simulink library "VIS_LIB"  (Simulink 8.6)
settings: Solver=ode45  StartTime=0.0  StopTime=10.0  RelTol=1e-3
undefined symbols (not defined in the file): AC, SIXOSEM_F_WD_AC_MASTER
libraries: cdsFilt x376, cdsEpicsOut x253, cdsEpicsIn x179, cdsTP x123, VIS_LIB x95, cdsMuxMatrix x91, cdsEpicsStringIn x75, cdsFiltCtrl x72, cdsFunctionCall x70, cdsRms x59, KAGRA_UTIL x25, STATE_BIO_MASTER x5
(part 1 of 38)
settings Model: Creator=keiko  LastModifiedBy=controls

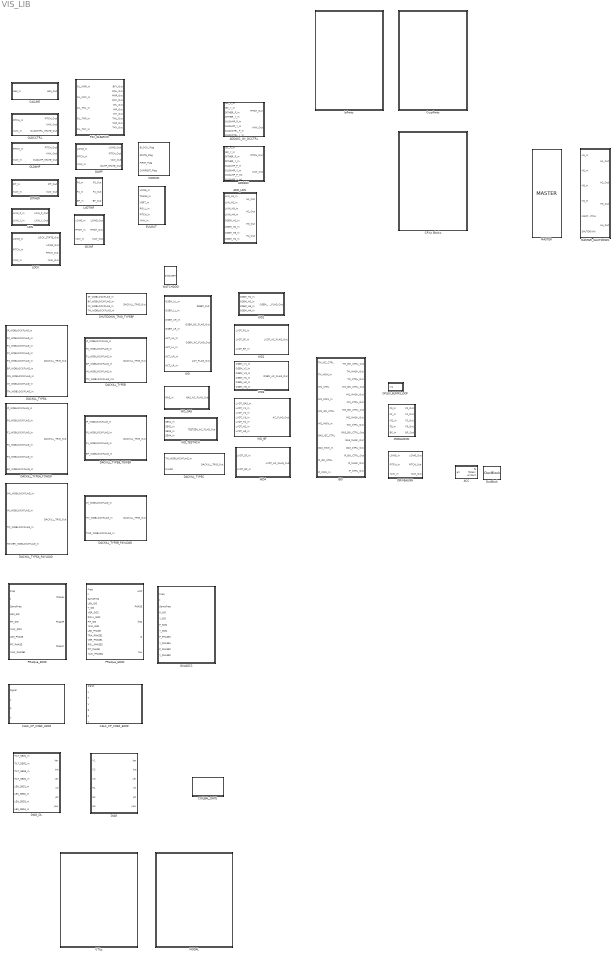
== system VIS_LIB ==
  ACC : Subsystem
  ADDASC : Subsystem
  ADDASC_W/_DCCTRL : Subsystem
  ADD_LKIN : Subsystem
  BIO : Subsystem
  CALC_CP_COEF_3DOF : Subsystem
  CALC_CP_COEF_6DOF : Subsystem
  CALLINE : Subsystem
  COILBAL_DATE : Subsystem
  CRYp Blocks : Subsystem
  CrypParts : Subsystem
  DACKILL_TYPEA : Subsystem
  DACKILL_TYPEA_PAYLOAD : Subsystem
  DACKILL_TYPEA_TOWER : Subsystem
  DACKILL_TYPEB : Subsystem
  DACKILL_TYPEB_PAYLOAD : Subsystem
  DACKILL_TYPEB_TOWER : Subsystem
  "DACKILL_TYPEC " : Subsystem
  DAMP : Subsystem
  DIAG : Subsystem
  DIAG_OL : Subsystem
  DITHER : Subsystem
  DRIVEALIGN : Subsystem
  DocBlock : simulink/Model-Wide Utilities/DocBlock  DocumentType=Text
  EULOUT : Subsystem
  ISCINF : Subsystem
  IpParts : Subsystem
  LKIN : Subsystem
  LOCK : Subsystem
  LVDTINF : Subsystem
  MASTER : CRYP_TM_MASTER/CRYP_TM_MASTER/MASTER
  MASTER_SHUTDOWN : Subsystem
  MODAL : Subsystem
  MODALMON : Subsystem
  OLDAMP : Subsystem
  OLDCCTRL : Subsystem
  OPLEV_BLRMS_DOF : Subsystem
  PAY_OLSERVO : Subsystem
  PReQua_3DOF : Subsystem
  PReQua_6DOF : Subsystem
  QUAASC1 : Subsystem
  SHUTDOWN_TRIG_TYPEBP : Subsystem
  UTILs : Subsystem
  WATCHDOG : cdsFunctionCall/Subsystem  Tag=cdsFunctionCall  Description=inline OSEMWATCHDOG $SUS_SRC/WATCHDOG.c
      settings: AttributesFormatString=%<Tag>\n%<Description>
  WD : Subsystem
  WD1 : Subsystem
  WD2 : Subsystem
  WD3 : Subsystem
  WD4 : Subsystem  AncestorBlock=VIS_LIB/WD2
  WDMON : Subsystem
  WD_BF : Subsystem
  WD_GAS : Subsystem
  WD_TEST4CH : Subsystem

== system VIS_LIB/ACC ==
  note: #DAQ Channels
      |
      | ACCSERVO_IN1 2048
      | ACCSERVO_OUT 2048
      | ERR2ACC_OUT 2048
      | FB2ACC_OUT 2048
  err : Inport
  ACCSERVO : cdsFilt/Subsystem  Tag=cdsFilt  Description=|
      | Purpose:                                                                                                                                                                                                                                  
      | Standard CDS IIR filter module.                                                                                                                                                                                                           
      |                                                                                                                                                                                                                                           
      | Operation:                                                                                                                                                                                                                                
      | Consists of 10 second order section IIR filters, plus a ramped gain stage. In FE code, also provides pre-defined test points and excitation channel inputs. The filter coefficients are defined in the LIGO system using the 'foton' tool.
      |                                                                                                                                                                                                                                           
      | Usage:                                                                                                                                                                                                                                    
      | Name the part with the desired filter module name.
      settings: AttributesFormatString=%<Tag>
  ERR2ACC : cdsFilt/Subsystem  Tag=cdsFilt  Description=|
      | Purpose:                                                                                                                                                                                                                                  
      | Standard CDS IIR filter module.                                                                                                                                                                                                           
      |                                                                                                                                                                                                                                           
      | Operation:                                                                                                                                                                                                                                
      | Consists of 10 second order section IIR filters, plus a ramped gain stage. In FE code, also provides pre-defined test points and excitation channel inputs. The filter coefficients are defined in the LIGO system using the 'foton' tool.
      |                                                                                                                                                                                                                                           
      | Usage:                                                                                                                                                                                                                                    
      | Name the part with the desired filter module name.
      settings: AttributesFormatString=%<Tag>
  FB2ACC : cdsFilt/Subsystem  Tag=cdsFilt  Description=|
      | Purpose:                                                                                                                                                                                                                                  
      | Standard CDS IIR filter module.                                                                                                                                                                                                           
      |                                                                                                                                                                                                                                           
      | Operation:                                                                                                                                                                                                                                
      | Consists of 10 second order section IIR filters, plus a ramped gain stage. In FE code, also provides pre-defined test points and excitation channel inputs. The filter coefficients are defined in the LIGO system using the 'foton' tool.
      |                                                                                                                                                                                                                                           
      | Usage:                                                                                                                                                                                                                                    
      | Name the part with the desired filter module name.
      settings: AttributesFormatString=%<Tag>
  fb : Outport
  fb2acc : Outport  Port=2
  err2acc : Outport  Port=3
  wires:
  ERR2ACC/1 -> err2acc/1
  FB2ACC/1 -> fb2acc/1
  ACCSERVO/1 -> FB2ACC/1, fb/1
  err/1 -> ACCSERVO/1, ERR2ACC/1

== system VIS_LIB/ADDASC ==
  ISC_P_In : Inport
  ISC_Y_In : Inport  Port=2
  DITHER_P_In : Inport  Port=3
  DITHER_Y_In : Inport  Port=4
  OLDAMP_P_In : Inport  Port=5
  OLDAMP_Y_In : Inport  Port=6
  OLDAMP_P_In2 : Inport  Port=7
  OLDAMP_Y_In1 : Inport  Port=8
  Sum3 : Sum  Inputs=++++
  Sum4 : Sum  Inputs=++++
  PITCH_Out : Outport
  YAW_Out : Outport  Port=2
  wires:
  DITHER_Y_In/1 -> Sum3/2
  DITHER_P_In/1 -> Sum4/2
  Sum4/1 -> PITCH_Out/1
  ISC_Y_In/1 -> Sum3/1
  ISC_P_In/1 -> Sum4/1
  Sum3/1 -> YAW_Out/1
  OLDAMP_P_In/1 -> Sum4/3
  OLDAMP_Y_In/1 -> Sum3/3
  OLDAMP_P_In2/1 -> Sum4/4
  OLDAMP_Y_In1/1 -> Sum3/4

== system VIS_LIB/ADDASC_W/_DCCTRL ==
  ISC_P_In : Inport
  ISC_Y_In : Inport  Port=2
  DITHER_P_In : Inport  Port=3
  DITHER_Y_In : Inport  Port=4
  OLDAMP_P_In : Inport  Port=5
  OLDAMP_Y_In : Inport  Port=6
  OLDCCTRL_P_In : Inport  Port=7
  OLDCCTRL_Y_In : Inport  Port=8
  Sum3 : Sum  Inputs=++++
  Sum4 : Sum  Inputs=++++
  PITCH_Out : Outport
  YAW_Out : Outport  Port=2
  wires:
  OLDAMP_Y_In/1 -> Sum3/3
  DITHER_Y_In/1 -> Sum3/2
  DITHER_P_In/1 -> Sum4/2
  OLDAMP_P_In/1 -> Sum4/3
  Sum4/1 -> PITCH_Out/1
  ISC_Y_In/1 -> Sum3/1
  ISC_P_In/1 -> Sum4/1
  Sum3/1 -> YAW_Out/1
  OLDCCTRL_P_In/1 -> Sum4/4
  OLDCCTRL_Y_In/1 -> Sum3/4

== system VIS_LIB/ADD_LKIN ==
  LKN_H1_In : Inport
  LKN_H2_In : Inport  Port=2
  LKIN_H3_In : Inport  Port=3
  LKIN_H4_In : Inport  Port=4
  OSEM_H1_In : Inport  Port=5
  OSEM_H2_In : Inport  Port=6
  OSEM_H3_In : Inport  Port=7
  OSEM_H4_In : Inport  Port=8
  Sum{,1,3..4} (4 alike) : Sum
  H1_Out : Outport
  H2_Out : Outport  Port=2
  H3_Out : Outport  Port=3
  H4_Out : Outport  Port=4
  wires:
  LKIN_H4_In/1 -> Sum1/1
  LKIN_H3_In/1 -> Sum3/1
  LKN_H2_In/1 -> Sum4/1
  Sum/1 -> H1_Out/1
  LKN_H1_In/1 -> Sum/1
  OSEM_H1_In/1 -> Sum/2
  Sum3/1 -> H3_Out/1
  Sum4/1 -> H2_Out/1
  OSEM_H3_In/1 -> Sum3/2
  OSEM_H2_In/1 -> Sum4/2
  Sum1/1 -> H4_Out/1
  OSEM_H4_In/1 -> Sum1/2

== system VIS_LIB/BIO ==
  note: 12 Bit Word
  note: 12 Bit Word
  note: 12 Bit Word
  note: 12 Bit Word
  TM_ISC_CTRL : Inport
  TM_MON_In : Inport  Port=2
  IM1_CTRL : Inport  Port=3
  IM1_MON_In : Inport  Port=4
  IM2_ISC_CTRL : Inport  Port=5
  IM2_MON_In : Inport  Port=6
  GAS_ISC_CTRL : Inport  Port=7
  GAS_MON_In : Inport  Port=8
  IP_ISC_CTRL : Inport  Port=9
  IP_MON_In : Inport  Port=10
  GAS : STATE_BIO_MASTER/UIM_BIO_MASTER
  IM1 : STATE_BIO_MASTER/UIM_BIO_MASTER
  IM2 : STATE_BIO_MASTER/UIM_BIO_MASTER
  IP : STATE_BIO_MASTER/TACQ_BIO_MASTER
  TM : STATE_BIO_MASTER/UIM_BIO_MASTER
  TM_BO_CTRL_Out : Outport
  TM_MASK_Out : Outport  Port=2
  TM_CTRL_Out : Outport  Port=3
  IM1_BO_CTRL_Out : Outport  Port=4
  IM1_MASK_Out : Outport  Port=5
  IM1_CTRL_Out : Outport  Port=6
  IM2_BO_CTRL_Out : Outport  Port=7
  IM2_MASK_Out : Outport  Port=8
  IM2_CTRL_Out : Outport  Port=9
  GAS_BO_CTRL_Out : Outport  Port=10
  GAS_MASK_Out : Outport  Port=11
  GAS_CTRL_Out : Outport  Port=12
  IP_BO_CTRL_Out : Outport  Port=13
  IP_MASK_Out : Outport  Port=14
  IP_CTRL_Out : Outport  Port=15
  wires:
  IP/3 -> IP_BO_CTRL_Out/1
  IP/2 -> IP_CTRL_Out/1
  IP/1 -> IP_MASK_Out/1
  GAS/3 -> GAS_BO_CTRL_Out/1
  GAS/2 -> GAS_CTRL_Out/1
  GAS/1 -> GAS_MASK_Out/1
  IM2/3 -> IM2_BO_CTRL_Out/1
  IM2/2 -> IM2_CTRL_Out/1
  IM2/1 -> IM2_MASK_Out/1
  IM1/3 -> IM1_BO_CTRL_Out/1
  IM1/2 -> IM1_CTRL_Out/1
  IM1/1 -> IM1_MASK_Out/1
  TM/3 -> TM_BO_CTRL_Out/1
  TM/2 -> TM_CTRL_Out/1
  TM/1 -> TM_MASK_Out/1
  IP_ISC_CTRL/1 -> IP/1
  IP_MON_In/1 -> IP/2
  GAS_ISC_CTRL/1 -> GAS/1
  GAS_MON_In/1 -> GAS/2
  IM2_ISC_CTRL/1 -> IM2/1
  IM2_MON_In/1 -> IM2/2
  IM1_MON_In/1 -> IM1/2
  IM1_CTRL/1 -> IM1/1
  TM_ISC_CTRL/1 -> TM/1
  TM_MON_In/1 -> TM/2

== system VIS_LIB/CALC_CP_COEF_3DOF ==
  Signal : Inport
  L : Inport  Port=2
  P : Inport  Port=3
  Y : Inport  Port=4
  BASE_SLCT : cdsMuxMatrix/Subsystem  Tag=cdsMuxMatrix  Description=Any size matrix. Inputs and outputs must be connected using Mux and Demux parts.
      settings: AttributesFormatString=%<Tag>
  COEF : cdsFilt/Subsystem  Tag=cdsFilt  Description=|
      | Purpose:                                                                                                                                                                                                                                  
      | Standard CDS IIR filter module.                                                                                                                                                                                                           
      |                                                                                                                                                                                                                                           
      | Operation:                                                                                                                                                                                                                                
      | Consists of 10 second order section IIR filters, plus a ramped gain stage. In FE code, also provides pre-defined test points and excitation channel inputs. The filter coefficients are defined in the LIGO system using the 'foton' tool.
      |                                                                                                                                                                                                                                           
      | Usage:                                                                                                                                                                                                                                    
      | Name the part with the desired filter module name.
      settings: AttributesFormatString=%<Tag>
  Demux1 : Demux  Outputs=1
  Divide : Product  Inputs=*/
  Mux1 : Mux  Inputs=3
  Terminator3 : Terminator
  wires:
  Y/1 -> Mux1/3
  BASE_SLCT/1 -> Demux1/1
  L/1 -> Mux1/1
  Demux1/1 -> Divide/2
  COEF/1 -> Terminator3/1
  Mux1/1 -> BASE_SLCT/1
  Signal/1 -> Divide/1
  Divide/1 -> COEF/1
  P/1 -> Mux1/2

== system VIS_LIB/CALC_CP_COEF_6DOF ==
  Signal : Inport
  L : Inport  Port=2
  T : Inport  Port=3
  V : Inport  Port=4
  R : Inport  Port=5
  P : Inport  Port=6
  Y : Inport  Port=7
  BASE_SLCT : cdsMuxMatrix/Subsystem  Tag=cdsMuxMatrix  Description=Any size matrix. Inputs and outputs must be connected using Mux and Demux parts.
      settings: AttributesFormatString=%<Tag>
  COEF : cdsFilt/Subsystem  Tag=cdsFilt  Description=|
      | Purpose:                                                                                                                                                                                                                                  
      | Standard CDS IIR filter module.                                                                                                                                                                                                           
      |                                                                                                                                                                                                                                           
      | Operation:                                                                                                                                                                                                                                
      | Consists of 10 second order section IIR filters, plus a ramped gain stage. In FE code, also provides pre-defined test points and excitation channel inputs. The filter coefficients are defined in the LIGO system using the 'foton' tool.
      |                                                                                                                                                                                                                                           
      | Usage:                                                                                                                                                                                                                                    
      | Name the part with the desired filter module name.
      settings: AttributesFormatString=%<Tag>
  Demux1 : Demux  Outputs=1
  Divide : Product  Inputs=*/
  Mux1 : Mux  Inputs=6
  wires:
  Divide/1 -> COEF/1
  Signal/1 -> Divide/1
  Mux1/1 -> BASE_SLCT/1
  Demux1/1 -> Divide/2
  BASE_SLCT/1 -> Demux1/1
  L/1 -> Mux1/1
  T/1 -> Mux1/2
  V/1 -> Mux1/3
  R/1 -> Mux1/4
  P/1 -> Mux1/5
  Y/1 -> Mux1/6

== system VIS_LIB/CALLINE ==
  LEN_In : Inport
  L : cdsFilt/Subsystem  Tag=cdsFilt  Description=|
      | Purpose:                                                                                                                                                                                                                                  
      | Standard CDS IIR filter module.                                                                                                                                                                                                           
      |                                                                                                                                                                                                                                           
      | Operation:                                                                                                                                                                                                                                
      | Consists of 10 second order section IIR filters, plus a ramped gain stage. In FE code, also provides pre-defined test points and excitation channel inputs. The filter coefficients are defined in the LIGO system using the 'foton' tool.
      |                                                                                                                                                                                                                                           
      | Usage:                                                                                                                                                                                                                                    
      | Name the part with the desired filter module name.
      settings: AttributesFormatString=%<Tag>
  LEN_Out : Outport
  wires:
  LEN_In/1 -> L/1
  L/1 -> LEN_Out/1

== system VIS_LIB/COILBAL_DATE ==
  DAY : cdsEpicsIn/Subsystem  Tag=cdsEpicsIn  Description=|
      | Purpose:                                                                              
      | Create an EPICS input channel connection to the FE realtime controls.                 
      |                                                                                       
      | Operation:                                                                            
      | Outputs value from an EPICS ai record. Value is floating point with a precision of 3..
      |                                                                                       
      | Usage:                                                                                
      | Name the part with the desired EPICS channel name.
      settings: AttributesFormatString=%<Tag>
  HOUR : cdsEpicsIn/Subsystem  Tag=cdsEpicsIn  Description=|
      | Purpose:                                                                              
      | Create an EPICS input channel connection to the FE realtime controls.                 
      |                                                                                       
      | Operation:                                                                            
      | Outputs value from an EPICS ai record. Value is floating point with a precision of 3..
      |                                                                                       
      | Usage:                                                                                
      | Name the part with the desired EPICS channel name.
      settings: AttributesFormatString=%<Tag>
  MIN : cdsEpicsIn/Subsystem  Tag=cdsEpicsIn  Description=|
      | Purpose:                                                                              
      | Create an EPICS input channel connection to the FE realtime controls.                 
      |                                                                                       
      | Operation:                                                                            
      | Outputs value from an EPICS ai record. Value is floating point with a precision of 3..
      |                                                                                       
      | Usage:                                                                                
      | Name the part with the desired EPICS channel name.
      settings: AttributesFormatString=%<Tag>
  MON : cdsEpicsIn/Subsystem  Tag=cdsEpicsIn  Description=|
      | Purpose:                                                                              
      | Create an EPICS input channel connection to the FE realtime controls.                 
      |                                                                                       
      | Operation:                                                                            
      | Outputs value from an EPICS ai record. Value is floating point with a precision of 3..
      |                                                                                       
      | Usage:                                                                                
      | Name the part with the desired EPICS channel name.
      settings: AttributesFormatString=%<Tag>
  Terminator{1..5} (5 alike) : Terminator
  YEAR : cdsEpicsIn/Subsystem  Tag=cdsEpicsIn  Description=|
      | Purpose:                                                                              
      | Create an EPICS input channel connection to the FE realtime controls.                 
      |                                                                                       
      | Operation:                                                                            
      | Outputs value from an EPICS ai record. Value is floating point with a precision of 3..
      |                                                                                       
      | Usage:                                                                                
      | Name the part with the desired EPICS channel name.
      settings: AttributesFormatString=%<Tag>
  wires:
  MIN/1 -> Terminator5/1
  DAY/1 -> Terminator3/1
  HOUR/1 -> Terminator4/1
  MON/1 -> Terminator2/1
  YEAR/1 -> Terminator1/1

== system VIS_LIB/CRYp Blocks ==
  COILOUTF : Subsystem
  MASTER : Subsystem
  PSWD : Subsystem

== system VIS_LIB/CrypParts ==
  ADD : Subsystem
  ADDALL : Subsystem
  ADDISC_IM : Subsystem
  ADDISC_MN : Subsystem
  ADDLOCAL_IM : Subsystem
  ADDLOCAL_MN : Subsystem
  ADD_TM : Subsystem
  DAMP : Subsystem
  DAMP_PY : Subsystem
  DRIVEALIGN : Subsystem
  LOCK : Subsystem
  OLDCCTRL : Subsystem
  OPLEV : Subsystem
  OPTICALIGN : Subsystem
  PSDAMP : Subsystem
  PSINF : Subsystem
  SUMOUT : Subsystem
  SUMOUT_TM : Subsystem
  TEST : Subsystem
  TEST_TM : Subsystem
  TM_OLSET : Subsystem

== system VIS_LIB/DACKILL_TYPEA ==
  note: WDBLOCKFLAG is zero (0) if OK,
      | non-zero if BAD
  note: AND is zero  (0) if all stages are OK
      | non-zero if BAD
  IP_WDBLOCKFLAG_In : Inport
  F0_WDBLOCKFLAG_In : Inport  Port=2
  F1_WDBLOCKFLAG_In : Inport  Port=3
  F2_WDBLOCKFLAG_In : Inport  Port=4
  F3_WDBLOCKFLAG_In : Inport  Port=5
  BF_WDBLOCKFLAG_In : Inport  Port=6
  MN_WDBLOCKFLAG_In : Inport  Port=7
  IM_WDBLOCKFLAG_In : Inport  Port=8
  TM_WDBLOCKFLAG_In : Inport  Port=9
  LogicalOperator1 : Logic  Operator=OR  Inputs=9  AllPortsSameDT=off  OutDataTypeStr=boolean
  STATE : cdsEpicsOut/Subsystem  Tag=cdsEpicsOutput  Description=|
      | Purpose:                                          
      | Output a FE signal to an EPICS channel.           
      |                                                   
      | Operation:                                        
      | Takes input value and passes it to EPICS record.  
      |                                                   
      | Usage:                                            
      | Name the part with the desired EPICS rrecord name.
      settings: AttributesFormatString=%<Tag>
  DACKILL_TRIG_Out : Outport
  wires:
  STATE/1 -> DACKILL_TRIG_Out/1
  IP_WDBLOCKFLAG_In/1 -> LogicalOperator1/1
  F0_WDBLOCKFLAG_In/1 -> LogicalOperator1/2
  F1_WDBLOCKFLAG_In/1 -> LogicalOperator1/3
  LogicalOperator1/1 -> STATE/1
  IM_WDBLOCKFLAG_In/1 -> LogicalOperator1/8
  BF_WDBLOCKFLAG_In/1 -> LogicalOperator1/6
  TM_WDBLOCKFLAG_In/1 -> LogicalOperator1/9
  MN_WDBLOCKFLAG_In/1 -> LogicalOperator1/7
  F3_WDBLOCKFLAG_In/1 -> LogicalOperator1/5
  F2_WDBLOCKFLAG_In/1 -> LogicalOperator1/4

== system VIS_LIB/DACKILL_TYPEA_PAYLOAD ==
  note: WDBLOCKFLAG is zero (0) if OK,
      | non-zero if BAD
  note: AND is zero  (0) if all stages are OK
      | non-zero if BAD
  MN_WDBLOCKFLAG_In : Inport
  IM_WDBLOCKFLAG_In : Inport  Port=2
  TM_WDBLOCKFLAG_In : Inport  Port=3
  TOWER_WDBLOCKFLAG_In : Inport  Port=4
  LogicalOperator1 : Logic  Operator=OR  Inputs=3  AllPortsSameDT=off  OutDataTypeStr=boolean
  LogicalOperator2 : Logic  Operator=OR  AllPortsSameDT=off  OutDataTypeStr=boolean
  PAYLOAD_STATE : cdsEpicsOut/Subsystem  Tag=cdsEpicsOutput  Description=|
      | Purpose:                                          
      | Output a FE signal to an EPICS channel.           
      |                                                   
      | Operation:                                        
      | Takes input value and passes it to EPICS record.  
      |                                                   
      | Usage:                                            
      | Name the part with the desired EPICS rrecord name.
      settings: AttributesFormatString=%<Tag>
  STATE : cdsEpicsOut/Subsystem  Tag=cdsEpicsOutput  Description=|
      | Purpose:                                          
      | Output a FE signal to an EPICS channel.           
      |                                                   
      | Operation:                                        
      | Takes input value and passes it to EPICS record.  
      |                                                   
      | Usage:                                            
      | Name the part with the desired EPICS rrecord name.
      settings: AttributesFormatString=%<Tag>
  DACKILL_TRIG_Out : Outport
  wires:
  LogicalOperator1/1 -> PAYLOAD_STATE/1
  IM_WDBLOCKFLAG_In/1 -> LogicalOperator1/2
  TM_WDBLOCKFLAG_In/1 -> LogicalOperator1/3
  MN_WDBLOCKFLAG_In/1 -> LogicalOperator1/1
  TOWER_WDBLOCKFLAG_In/1 -> LogicalOperator2/2
  PAYLOAD_STATE/1 -> LogicalOperator2/1
  LogicalOperator2/1 -> STATE/1
  STATE/1 -> DACKILL_TRIG_Out/1

== system VIS_LIB/DACKILL_TYPEA_TOWER ==
  note: WDBLOCKFLAG is zero (0) if OK,
      | non-zero if BAD
  note: AND is zero  (0) if all stages are OK
      | non-zero if BAD
  IP_WDBLOCKFLAG_In : Inport
  F0_WDBLOCKFLAG_In : Inport  Port=2
  F1_WDBLOCKFLAG_In : Inport  Port=3
  F2_WDBLOCKFLAG_In : Inport  Port=4
  F3_WDBLOCKFLAG_In : Inport  Port=5
  BF_WDBLOCKFLAG_In : Inport  Port=6
  LogicalOperator1 : Logic  Operator=OR  Inputs=6  AllPortsSameDT=off  OutDataTypeStr=boolean
  STATE : cdsEpicsOut/Subsystem  Tag=cdsEpicsOutput  Description=|
      | Purpose:                                          
      | Output a FE signal to an EPICS channel.           
      |                                                   
      | Operation:                                        
      | Takes input value and passes it to EPICS record.  
      |                                                   
      | Usage:                                            
      | Name the part with the desired EPICS rrecord name.
      settings: AttributesFormatString=%<Tag>
  DACKILL_TRIG_Out : Outport
  wires:
  STATE/1 -> DACKILL_TRIG_Out/1
  IP_WDBLOCKFLAG_In/1 -> LogicalOperator1/1
  F0_WDBLOCKFLAG_In/1 -> LogicalOperator1/2
  F1_WDBLOCKFLAG_In/1 -> LogicalOperator1/3
  LogicalOperator1/1 -> STATE/1
  BF_WDBLOCKFLAG_In/1 -> LogicalOperator1/6
  F3_WDBLOCKFLAG_In/1 -> LogicalOperator1/5
  F2_WDBLOCKFLAG_In/1 -> LogicalOperator1/4

== system VIS_LIB/DACKILL_TYPEB ==
  note: WDBLOCKFLAG is zero (0) if OK,
      | non-zero if BAD
  note: AND is zero  (0) if all stages are OK
      | non-zero if BAD
  IP_WDBLOCKFLAG_In : Inport
  F0_WDBLOCKFLAG_In : Inport  Port=2
  F1_WDBLOCKFLAG_In : Inport  Port=3
  BF_WDBLOCKFLAG_In : Inport  Port=4
  IM_WDBLOCKFLAG_In : Inport  Port=5
  TM_WDBLOCKFLAG_In1 : Inport  Port=6
  LogicalOperator1 : Logic  Operator=OR  Inputs=6  AllPortsSameDT=off  OutDataTypeStr=boolean
  STATE : cdsEpicsOut/Subsystem  Tag=cdsEpicsOutput  Description=|
      | Purpose:                                          
      | Output a FE signal to an EPICS channel.           
      |                                                   
      | Operation:                                        
      | Takes input value and passes it to EPICS record.  
      |                                                   
      | Usage:                                            
      | Name the part with the desired EPICS rrecord name.
      settings: AttributesFormatString=%<Tag>
  DACKILL_TRIG_Out : Outport
  wires:
  STATE/1 -> DACKILL_TRIG_Out/1
  IP_WDBLOCKFLAG_In/1 -> LogicalOperator1/1
  F0_WDBLOCKFLAG_In/1 -> LogicalOperator1/2
  F1_WDBLOCKFLAG_In/1 -> LogicalOperator1/3
  LogicalOperator1/1 -> STATE/1
  IM_WDBLOCKFLAG_In/1 -> LogicalOperator1/5
  BF_WDBLOCKFLAG_In/1 -> LogicalOperator1/4
  TM_WDBLOCKFLAG_In1/1 -> LogicalOperator1/6

== system VIS_LIB/DACKILL_TYPEB_PAYLOAD ==
  note: WDBLOCKFLAG is zero (0) if OK,
      | non-zero if BAD
  note: AND is zero  (0) if all stages are OK
      | non-zero if BAD
  IM_WDBLOCKFLAG_In : Inport
  TM_WDBLOCKFLAG_In : Inport  Port=2
  TWR_WDBLOCKFLAG_In : Inport  Port=3
  LogicalOperator1 : Logic  Operator=OR  Inputs=3  AllPortsSameDT=off  OutDataTypeStr=boolean
  STATE : cdsEpicsOut/Subsystem  Tag=cdsEpicsOutput  Description=|
      | Purpose:                                          
      | Output a FE signal to an EPICS channel.           
      |                                                   
      | Operation:                                        
      | Takes input value and passes it to EPICS record.  
      |                                                   
      | Usage:                                            
      | Name the part with the desired EPICS rrecord name.
      settings: AttributesFormatString=%<Tag>
  DACKILL_TRIG_Out : Outport
  wires:
  STATE/1 -> DACKILL_TRIG_Out/1
  LogicalOperator1/1 -> STATE/1
  IM_WDBLOCKFLAG_In/1 -> LogicalOperator1/1
  TM_WDBLOCKFLAG_In/1 -> LogicalOperator1/2
  TWR_WDBLOCKFLAG_In/1 -> LogicalOperator1/3

== system VIS_LIB/DACKILL_TYPEB_TOWER ==
  note: WDBLOCKFLAG is zero (0) if OK,
      | non-zero if BAD
  note: AND is zero  (0) if all stages are OK
      | non-zero if BAD
  IP_WDBLOCKFLAG_In : Inport
  F0_WDBLOCKFLAG_In : Inport  Port=2
  F1_WDBLOCKFLAG_In : Inport  Port=3
  BF_WDBLOCKFLAG_In : Inport  Port=4
  LogicalOperator1 : Logic  Operator=OR  Inputs=4  AllPortsSameDT=off  OutDataTypeStr=boolean
  STATE : cdsEpicsOut/Subsystem  Tag=cdsEpicsOutput  Description=|
      | Purpose:                                          
      | Output a FE signal to an EPICS channel.           
      |                                                   
      | Operation:                                        
      | Takes input value and passes it to EPICS record.  
      |                                                   
      | Usage:                                            
      | Name the part with the desired EPICS rrecord name.
      settings: AttributesFormatString=%<Tag>
  DACKILL_TRIG_Out : Outport
  wires:
  STATE/1 -> DACKILL_TRIG_Out/1
  IP_WDBLOCKFLAG_In/1 -> LogicalOperator1/1
  F0_WDBLOCKFLAG_In/1 -> LogicalOperator1/2
  F1_WDBLOCKFLAG_In/1 -> LogicalOperator1/3
  LogicalOperator1/1 -> STATE/1
  BF_WDBLOCKFLAG_In/1 -> LogicalOperator1/4

== system VIS_LIB/DACKILL_TYPEC  ==
  note: WDBLOCKFLAG is zero (0) if OK,
      | non-zero if BAD
  note: AND is zero  (0) if all stages are OK
      | non-zero if BAD
  TM_WDBLOCKFLAG_In : Inport
  FLAG0 : Inport  Port=2
  LogicalOperator1 : Logic  Operator=OR  AllPortsSameDT=off  OutDataTypeStr=boolean
  STATE : cdsEpicsOut/Subsystem  Tag=cdsEpicsOutput  Description=|
      | Purpose:                                          
      | Output a FE signal to an EPICS channel.           
      |                                                   
      | Operation:                                        
      | Takes input value and passes it to EPICS record.  
      |                                                   
      | Usage:                                            
      | Name the part with the desired EPICS rrecord name.
      settings: AttributesFormatString=%<Tag>
  DACKILL_TRIG_Out : Outport
  wires:
  STATE/1 -> DACKILL_TRIG_Out/1
  TM_WDBLOCKFLAG_In/1 -> LogicalOperator1/2
  LogicalOperator1/1 -> STATE/1
  FLAG0/1 -> LogicalOperator1/1
